simulink model "linProg_test"  (R2017a)
settings: Solver=VariableStepAuto  StartTime=0.0  StopTime=.1  RelTol=1e-3
settings Model: Creator=erich  LastModifiedBy=erich

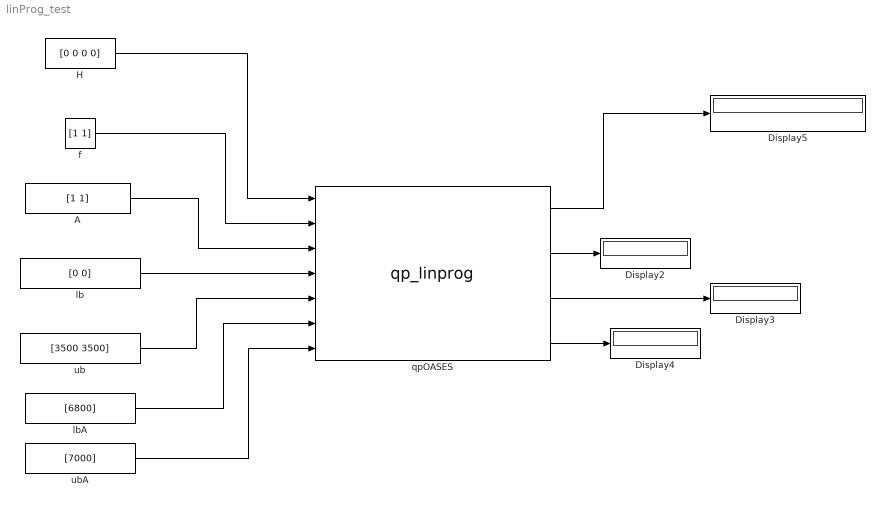
== system linProg_test ==
  A : Constant  Value=[1 1]  VectorParams1D=off
  Display{2..5} (4 alike) : Display
  H : Constant  Value=[0 0 0 0]
  f : Constant  Value=[1 1]
  lb : Constant  Value=[0 0]
  lbA : Constant  Value=[6800]
  qpOASES : S-Function  FunctionName=qp_linprog  SFunctionDeploymentMode=off  EnableBusSupport=off
  ub : Constant  Value=[3500 3500]
  ubA : Constant  Value=[7000]
  wires:
  qpOASES/1 -> Display5/1
  H/1 -> qpOASES/1
  f/1 -> qpOASES/2
  A/1 -> qpOASES/3
  lb/1 -> qpOASES/4
  ub/1 -> qpOASES/5
  lbA/1 -> qpOASES/6
  ubA/1 -> qpOASES/7
  qpOASES/2 -> Display2/1
  qpOASES/3 -> Display3/1
  qpOASES/4 -> Display4/1
